simulink model "case_5_lead_car_appears25a"  (R2025b)
settings: Solver=VariableStepAuto  StartTime=0.0  StopTime=10.0  RelTol=1e-3
settings Model: Creator=jdcjd  LastModifiedBy=admin

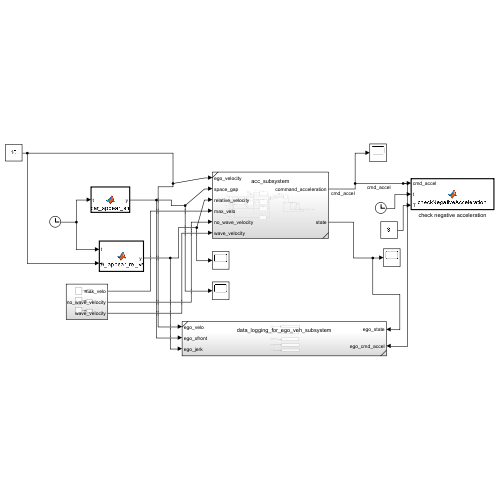
[thumbnail: Simulink's stored preview of the top-level diagram]
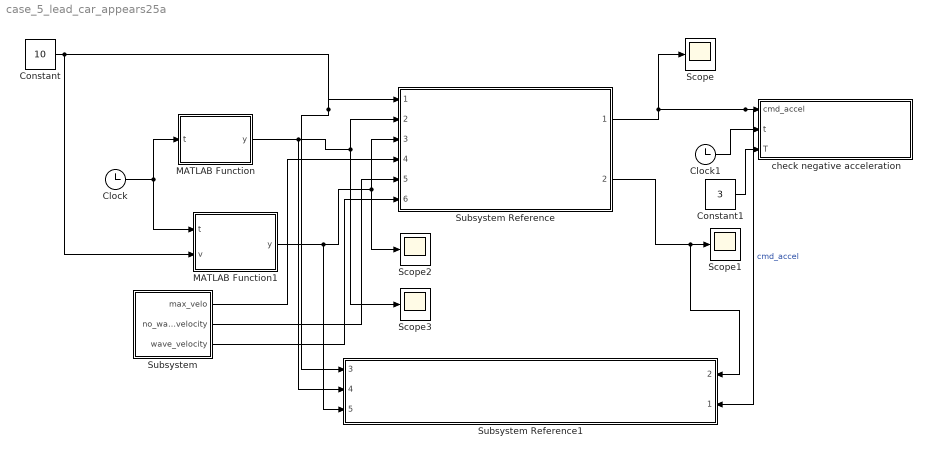
== system case_5_lead_car_appears25a ==
  Clock : Clock
  Clock1 : Clock
  Constant : Constant  Value=10
  Constant1 : Constant  Value=3
  MATLAB Function : MATLAB Function  TreatAsAtomicUnit=on
  MATLAB Function1 : MATLAB Function  TreatAsAtomicUnit=on
  Scope{,1..3} (4 alike) : Scope
      Scope settings: ActiveDisplayYMinimum=-3.5625  ActiveDisplayYMaximum=2.0625
      Scope2 settings: ActiveDisplayYMinimum=2.5000000000000018  ActiveDisplayYMaximum=77.5  DataLoggingVariableName=ScopeData2
      Scope3 settings: ActiveDisplayYMinimum=4.3537066340928323  ActiveDisplayYMaximum=25.005048531522391  DataLoggingVariableName=ScopeData3
  Subsystem : Subsystem
  Subsystem Reference : Subsystem  ReferencedSubsystem=acc_subsystem
  Subsystem Reference1 : Subsystem  ReferencedSubsystem=data_logging_for_ego_veh_subsystem
      settings: PortSchema="{\"entries\":[{\"content\":{\"sides\":[{\"content\":{\"connectorIds\":[\"In3\",\"In4\",\"In5\"]},\"type\":\"ConnectorPlacement.EquallySpacedRectSide\",\"uuid\":\"0b96bcaa-a470-46c9-9268-f4bd6b1035a8\"},{\"content\":{\"connectorIds\":[\"In2\",\"In1\"],\"side\":\"RIGHT\"},\"type\":\"ConnectorPlacement.EquallySpacedRectSide\",\"uuid\":\"8e49005a-1e53-4e76-b163-50df0eb9f2cc\"},{\"content\":{\"side\":\"TOP\"},\"type\":\"ConnectorPlacement.EquallySpacedRectSide\",\"uuid\":\"3ff4af65-efca-4a64-9b7f-f479498e89e2\"}]},\"type\":\"ConnectorPlacement.EquallySpacedConnector\",\"uuid\":\"f10caef7-9599-4d5c-a8fd-3eb49f6fcaa8\"}],\"packageUris\":[\"http://schema.mathworks.com/mf0/Connector/R2020b\"],\"version\":\"1.0\"}"
  check negative acceleration : MATLAB Function  TreatAsAtomicUnit=on
  wires:
  Constant/1 -> Subsystem Reference1/3, Subsystem Reference/1, MATLAB Function1/2(v)
  Clock/1 -> MATLAB Function/1(t), MATLAB Function1/1(t)
  MATLAB Function/1(y) -> Subsystem Reference1/4, Scope3/1, Subsystem Reference/2
  Constant1/1 -> check negative acceleration/3(T)
  Clock1/1 -> check negative acceleration/2(t)
  Subsystem Reference/1 -> Scope/1, Subsystem Reference1/1, check negative acceleration/1(cmd_accel)  "cmd_accel"
  Subsystem Reference/2 -> Subsystem Reference1/2, Scope1/1
  MATLAB Function1/1(y) -> Scope2/1, Subsystem Reference/3, Subsystem Reference1/5
  Subsystem/1(max_velo) -> Subsystem Reference/4
  Subsystem/2(no_wave_velocity) -> Subsystem Reference/5
  Subsystem/3(wave_velocity) -> Subsystem Reference/6

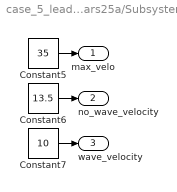
== system case_5_lead_car_appears25a/Subsystem ==
  Constant5 : Constant  Value=35
  Constant6 : Constant  Value=13.5
  Constant7 : Constant  Value=10
  max_velo : Outport
  no_wave_velocity : Outport  Port=2
  wave_velocity : Outport  Port=3
  wires:
  Constant7/1 -> wave_velocity/1
  Constant6/1 -> no_wave_velocity/1
  Constant5/1 -> max_velo/1

== matlab function case_5_lead_car_appears25a/MATLAB Function ==
  data: t input; y output
function y = car_appear_sn(t)

if t < 3
    y = inf;
else
    y = 15;
end
end

== matlab function case_5_lead_car_appears25a/check negative acceleration ==
  data: cmd_accel input; t input; T input
function checkNegativeAcceleration(cmd_accel, t, T)
%#codegen
coder.extrinsic('disp', 'sprintf');

if (cmd_accel >= 0) && (t>T)
    msg = sprintf('Error: Positive command acceleration: %.3f, should be negative', ...
                  cmd_accel);
    disp(msg);
end
end

== matlab function case_5_lead_car_appears25a/MATLAB Function1 ==
  data: t input; y output; v input
function y = car_appear_rel_vel(t, v)

if t < 3
    y =v;
else 
    y = 8*t -v;
end
end
